simulink subsystem "Day3_Scenario_1"  (R2024a)
settings: Solver=VariableStepAuto  StartTime=0.0  StopTime=10.0  RelTol=1e-3
undefined symbols (not defined in the file): left_first_line_point_x, right_first_line_point_x
libraries: CarMaker4SL x6, slpidlib x1
settings Model: Creator=junhyung.cha  LastModifiedBy=User

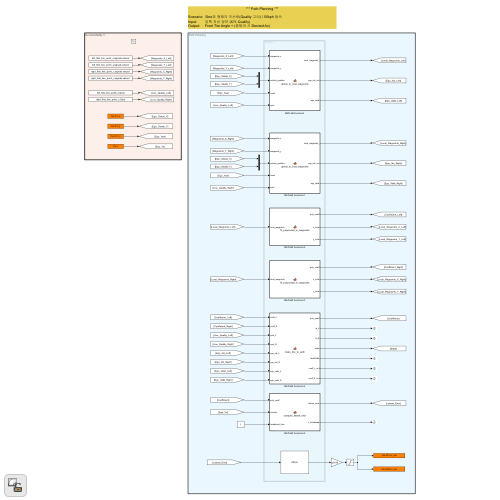
[thumbnail: Simulink's stored preview of the top-level diagram]
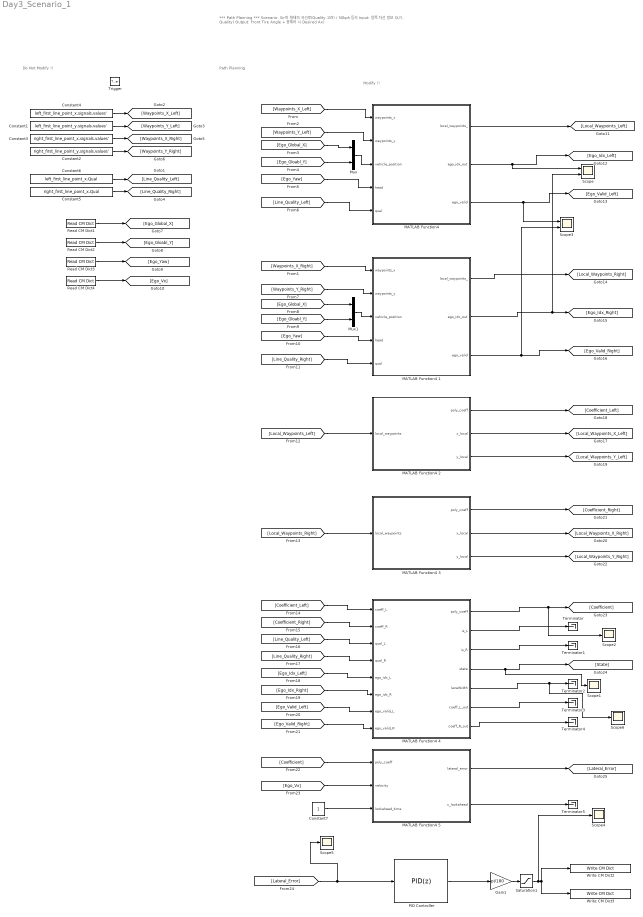
== system Day3_Scenario_1 ==
  note: Path Planning
  note: Do Not Modify !!
  note: Modify !!
  note: *** Path Planning ***
      |
      | Scenario: Sine파 형태의 곡선로(Quality 고려) / 50kph 등속
      | Input: 양쪽 차선 정보 (X/Y, Quality)
      | Output: Front Tire Angle + (종제어 시 Desired Ax)
  Trigger : TriggerPort  TriggerType=function-call  VariantControl=(inherit)
  Constant1 : Constant  Value=left_first_line_point_y.signals.values'
  Constant2 : Constant  Value=right_first_line_point_y.signals.values'
  Constant3 : Constant  Value=right_first_line_point_x.signals.values'
  Constant4 : Constant  Value=left_first_line_point_x.signals.values'
  Constant5 : Constant  Value=right_first_line_point_x.Qual
  Constant6 : Constant  Value=left_first_line_point_x.Qual
  Constant7 : Constant
  Gain1 : Gain  Gain=pi/180
  "MATLAB Function4 " : MATLAB Function  TreatAsAtomicUnit=on
  MATLAB Function4 1 : MATLAB Function  TreatAsAtomicUnit=on
  MATLAB Function4 2 : MATLAB Function  TreatAsAtomicUnit=on
  MATLAB Function4 3 : MATLAB Function  TreatAsAtomicUnit=on
  MATLAB Function4 4 : MATLAB Function  TreatAsAtomicUnit=on
  MATLAB Function4 5 : MATLAB Function  TreatAsAtomicUnit=on
  Mux : Mux  Inputs=2
  Mux1 : Mux  Inputs=2
  PID Controller : slpidlib/PID Controller  Controller=PID  Form=Parallel  TimeDomain=Discrete-time  UseExternalTs=off  SampleTime=-1  IntegratorMethod=Forward Euler  FilterMethod=Forward Euler  ControllerParametersSource=internal  P=0.2  I=0  UseKiTs=off  D=0.0001  UseExternalDerivativeSource=off  N=100  UseFilter=off  TunerSelectOption=Transfer Function Based (PID Tuner App)  InitialConditionSource=internal  InitialConditionForIntegrator=0  InitialConditionForFilter=0  DifferentiatorICPrevScaledInput=0  ExternalReset=none  TrackingMode=off  Kt=1  LimitOutput=off  SatLimitsSource=internal  UpperSaturationLimit=inf  LowerSaturationLimit=-inf  LinearizeAsGain=on  AntiWindupMode=none  Kb=1  LimitIntegrator=off  UpperIntegratorSaturationLimit=inf  LowerIntegratorSaturationLimit=-inf  POutMin=[]  POutMax=[]  IOutMin=[]  IOutMax=[]  DOutMin=[]  DOutMax=[]  NOutMin=[]  NOutMax=[]  SumOutMin=[]  SumOutMax=[]  SaturationOutMin=[]  SaturationOutMax=[]  PParamMin=[]  PParamMax=[]  IParamMin=[]  IParamMax=[]  DParamMin=[]  DParamMax=[]  NParamMin=[]  NParamMax=[]  KbParamMin=[]  KbParamMax=[]  KtParamMin=[]  KtParamMax=[]  KbOutMin=[]  KbOutMax=[]  KtOutMin=[]  KtOutMax=[]  IntegratorOutMin=[]  IntegratorOutMax=[]  FilterOutMin=[]  FilterOutMax=[]  SumI1OutMin=[]  SumI1OutMax=[]  SumI2OutMin=[]  SumI2OutMax=[]  SumI3OutMin=[]  SumI3OutMax=[]  SumI4OutMin=[]  SumI4OutMax=[]  SumDOutMin=[]  SumDOutMax=[]  DifferentiatorOutMin=[]  DifferentiatorOutMax=[]  FilterDiffOutCoefMin=[]  FilterDiffOutCoefMax=[]  ReciprocalOutMin=[]  ReciprocalOutMax=[]  SumDenOutMin=[]  SumDenOutMax=[]  SumNumOutMin=[]  SumNumOutMax=[]  DivideOutMin=[]  DivideOutMax=[]  UdiffTsProdOutMin=[]  UdiffTsProdOutMax=[]  NTsProdOutMin=[]  NTsProdOutMax=[]  UintegralTsProdOutMin=[]  UintegralTsProdOutMax=[]  UngainTsProdOutMin=[]  UngainTsProdOutMax=[]  ClampingZeroOutDataTypeStr=Inherit: Inherit via back propagation  ClampingZeroOutMin=[]  ClampingZeroOutMax=[]  FilterDenConstantOutDataTypeStr=Inherit: Inherit via back propagation  FilterDenConstantOutMin=[]  FilterDenConstantOutMax=[]  PCopyOutDataTypeStr=Inherit: Inherit via back propagation  PCopyOutMin=[]  PCopyOutMax=[]  NCopyOutDataTypeStr=Inherit: Inherit via back propagation  NCopyOutMin=[]  NCopyOutMax=[]  IntegratorContinuousStateAttributes=''  IntegratorStateMustResolveToSignalObject=off  IntegratorRTWStateStorageClass=Auto  FilterContinuousStateAttributes=''  FilterStateMustResolveToSignalObject=off  FilterRTWStateStorageClass=Auto  ParallelPVariant=InternalParameters  IdealPVariant=Disabled  IVariant=InternalParameters  DVariant=InternalParameters  IntegratorVariant=Discrete  SatVariant=Disabled  AWVariant=Passthrough  PCopyVariant=Disabled  TRVariant=Disabled  FdbkBlocksVariant=Forward  IdealPFdbkVariant=Disabled  SatFdbkVariant=Disabled  DerivativeFilterVariant=Differentiator  NVariant=Passthrough  NCopyVariant=Disabled_SignalSpec  FilterICVariant=InternalICsDifferentiator  IntegratorICVariant=InternalICs  ExternalResetVariant=Disabled  TRSumVariant=Passthrough  SumFdbkVariant=Disabled  SumVariant=Sum_PID  TsampFilterVariant=InternalTs  TsampNgainVariant=Passthrough  TsampIntegralVariant=Disabled_SignalSpec  ExternalSaturationOutDataTypeStr=Inherit: Same as second input  DerivativeSourceVariant=ErrorSignal
  Read CM Dict1 : CarMaker4SL/Read CM Dict  xname=Car.Fr1.tx  xsync=off  xstime=Inherited
  Read CM Dict2 : CarMaker4SL/Read CM Dict  xname=Car.Fr1.ty  xsync=off  xstime=Inherited
  Read CM Dict3 : CarMaker4SL/Read CM Dict  xname=Car.Fr1.rz  xsync=off  xstime=Inherited
  Read CM Dict4 : CarMaker4SL/Read CM Dict  xname=Car.v  xsync=off  xstime=Inherited
  Saturation1 : Saturate  UpperLimit=2  LowerLimit=-2
  Scope : Scope  NumInputPorts=2
  Scope{1..2,4..6} (5 alike) : Scope
  Scope3 : Scope  NumInputPorts=2
  Terminator{,1..5} (6 alike) : Terminator
  Write CM Dict2 : CarMaker4SL/Write CM Dict  xname=Car.CFL.rz_ext  xsync=off
  Write CM Dict3 : CarMaker4SL/Write CM Dict  xname=Car.CFR.rz_ext  xsync=off
  wires:
  Constant4/1 -> [Waypoints_X_Left]
  Constant1/1 -> [Waypoints_Y_Left]
  Constant2/1 -> [Waypoints_Y_Right]
  Constant3/1 -> [Waypoints_X_Right]
  [Waypoints_X_Left] -> "MATLAB Function4 "/1(waypoints_x)
  [Waypoints_Y_Left] -> "MATLAB Function4 "/2(waypoints_y)
  Mux/1 -> "MATLAB Function4 "/3(vehicle_position)
  [Ego_Global_X] -> Mux/1
  Read CM Dict2/1 -> [Ego_Gloabl_Y]
  Read CM Dict1/1 -> [Ego_Global_X]
  [Ego_Gloabl_Y] -> Mux/2
  Read CM Dict3/1 -> [Ego_Yaw]
  [Ego_Yaw] -> "MATLAB Function4 "/4(head)
  Constant5/1 -> [Line_Quality_Right]
  Constant6/1 -> [Line_Quality_Left]
  [Line_Quality_Right] -> MATLAB Function4 1/5(qual)
  [Ego_Yaw] -> MATLAB Function4 1/4(head)
  [Ego_Gloabl_Y] -> Mux1/2
  [Ego_Global_X] -> Mux1/1
  [Waypoints_Y_Right] -> MATLAB Function4 1/2(waypoints_y)
  [Waypoints_X_Right] -> MATLAB Function4 1/1(waypoints_x)
  Mux1/1 -> MATLAB Function4 1/3(vehicle_position)
  "MATLAB Function4 "/3(ego_valid) -> [Ego_Valid_Left], Scope3/1
  "MATLAB Function4 "/2(ego_idx_out) -> [Ego_Idx_Left], Scope/1
  "MATLAB Function4 "/1(local_waypoints_) -> [Local_Waypoints_Left]
  MATLAB Function4 1/1(local_waypoints_) -> [Local_Waypoints_Right]
  MATLAB Function4 1/2(ego_idx_out) -> [Ego_Idx_Right], Scope/2
  MATLAB Function4 1/3(ego_valid) -> [Ego_Valid_Right], Scope3/2
  [Local_Waypoints_Left] -> MATLAB Function4 2/1(local_waypoints)
  [Local_Waypoints_Right] -> MATLAB Function4 3/1(local_waypoints)
  MATLAB Function4 2/1(poly_coeff) -> [Coefficient_Left]
  MATLAB Function4 2/2(x_local) -> [Local_Waypoints_X_Left]
  MATLAB Function4 2/3(y_local) -> [Local_Waypoints_Y_Left]
  MATLAB Function4 3/3(y_local) -> [Local_Waypoints_Y_Right]
  MATLAB Function4 3/2(x_local) -> [Local_Waypoints_X_Right]
  MATLAB Function4 3/1(poly_coeff) -> [Coefficient_Right]
  [Coefficient_Left] -> MATLAB Function4 4/1(coeff_L)
  [Line_Quality_Left] -> MATLAB Function4 4/3(qual_L)
  [Ego_Idx_Left] -> MATLAB Function4 4/5(ego_idx_L)
  [Ego_Idx_Right] -> MATLAB Function4 4/6(ego_idx_R)
  [Ego_Valid_Left] -> MATLAB Function4 4/7(ego_valid_L)
  [Ego_Valid_Right] -> MATLAB Function4 4/8(ego_valid_R)
  MATLAB Function4 4/1(poly_coeff) -> [Coefficient], Scope2/1
  MATLAB Function4 4/4(state) -> [State], Scope1/1
  MATLAB Function4 4/2(is_L) -> Terminator/1
  MATLAB Function4 4/3(is_R) -> Terminator1/1
  MATLAB Function4 4/6(coeff_L_out) -> Terminator3/1
  MATLAB Function4 4/5(laneWidth) -> Terminator2/1, Scope6/1
  MATLAB Function4 4/7(coeff_R_out) -> Terminator4/1
  [Coefficient] -> MATLAB Function4 5/1(poly_coeff)
  Read CM Dict4/1 -> [Ego_Vx]
  [Ego_Vx] -> MATLAB Function4 5/2(velocity)
  Constant7/1 -> MATLAB Function4 5/3(lookahead_time)
  Saturation1/1 -> Write CM Dict3/1, Write CM Dict2/1, Scope4/1
  Gain1/1 -> Saturation1/1
  MATLAB Function4 5/1(lateral_error) -> [Lateral_Error]
  MATLAB Function4 5/2(x_lookahead) -> Terminator5/1
  [Lateral_Error] -> PID Controller/1, Scope5/1
  PID Controller/1 -> Gain1/1
  [Line_Quality_Left] -> "MATLAB Function4 "/5(qual)
  [Coefficient_Right] -> MATLAB Function4 4/2(coeff_R)
  [Line_Quality_Right] -> MATLAB Function4 4/4(qual_R)

== matlab function Day3_Scenario_1/MATLAB Function4 5 ==
  settings: sampleTime=0.1
  data: poly_coeff input; lateral_error output; x_lookahead output; velocity input; lookahead_time input
function [lateral_error, x_lookahead] = compute_lateral_error(poly_coeff, velocity, lookahead_time)
%#codegen
% compute_lateral_error - Look-ahead 지점에서의 lateral error 계산
%   poly_coeff     : 1x4 다항식 계수 [a3 a2 a1 a0]
%   velocity       : 차량 전진 속도 (m/s)
%   lookahead_time : look-ahead 시간 (s)
%
% 출력:
%   lateral_error  : lateral error + heading error 보정값
%   x_lookahead    : look-ahead 거리

    %% 1) lookahead 거리
    x_lookahead = velocity * lookahead_time;

    %% 2) 경로상의 y 위치
    y = polyval(poly_coeff, x_lookahead);

    %% 3) 경로 기울기 → 방향 각도
    dpoly = polyder(poly_coeff);
    dy_dx = polyval(dpoly, x_lookahead);
    path_theta = atan(dy_dx);

    %% 4) heading error (차량 방향 θ_vehicle = 0 가정)
    heading_error = path_theta;

    %% 5) lateral error 보정 (tunable gain)
    k_heading = 1.0;  
    lateral_error = y + k_heading * heading_error;
     %% 6) lateral error 클리핑 (안정성 확보)
    max_error = 10.0;  % 필요시 조절
    lateral_error = min(max(lateral_error, -max_error), max_error);
end

== matlab function Day3_Scenario_1/MATLAB Function4  ==
  settings: sampleTime=0.1
  data: waypoints_x input; waypoints_y input; local_waypoints_ output; vehicle_position input; head input; ego_idx_out output; ego_valid output; qual input
function [local_waypoints_, ego_idx_out, ego_valid] = global_to_local_waypoints_left(waypoints_x, waypoints_y, vehicle_position, head, qual)
    % 우측 차선 전역 → 로컬 좌표 변환 및 유효 인덱스 계산

    N = numel(waypoints_x);
    local_waypoints_ = zeros(N, 2);

    % 차량 yaw 방향의 회전 행렬 파라미터
    cos_h = cos(head);
    sin_h = sin(head);

    % 1) 전역 좌표 → 로컬 좌표
    for i = 1:N
        dx = waypoints_x(i) - vehicle_position(1);
        dy = waypoints_y(i) - vehicle_position(2);
        % (x', y') = R(-head) * [dx; dy]
        x_local =  dx * cos_h + dy * sin_h;
        y_local = -dx * sin_h + dy * cos_h;
        local_waypoints_(i, :) = [x_local, y_local];
    end

    % 2) qual == 1 (유효)인 인덱스들만 추출
    valid_indices = find(qual == 1);

    % 파라미터: 최대 인식 거리
    max_distance = 30; % meter

    % 3) 유효 지점 중 전방 x_local 거리 기준 최소값 선택 (30m 이내만)
    if ~isempty(valid_indices)
        x_vals = local_waypoints_(valid_indices, 1);
        d_vals = abs(x_vals);  % 전방 거리 기준
        d_vals(x_vals < 0 | d_vals > max_distance) = Inf;  % 후방 또는 너무 먼 점 제거

        [~, idx_min] = min(d_vals);
        if isinf(d_vals(idx_min))
            ego_idx_out = -1;
            ego_valid   = 0;
        else
            ego_idx_out = valid_indices(idx_min);
            ego_valid   = 1;
        end
    else
        ego_idx_out = -1;
        ego_valid   = 0;
    end
end

== matlab function Day3_Scenario_1/MATLAB Function4 1 ==
  settings: sampleTime=0.1
  data: waypoints_x input; waypoints_y input; local_waypoints_ output; vehicle_position input; head input; qual input; ego_idx_out output; ego_valid output
function [local_waypoints_, ego_idx_out, ego_valid] = global_to_local_waypoints_left(waypoints_x, waypoints_y, vehicle_position, head, qual)
    % 우측 차선 전역 → 로컬 좌표 변환 및 유효 인덱스 계산

    N = numel(waypoints_x);
    local_waypoints_ = zeros(N, 2);

    % 차량 yaw 방향의 회전 행렬 파라미터
    cos_h = cos(head);
    sin_h = sin(head);

    % 1) 전역 좌표 → 로컬 좌표
    for i = 1:N
        dx = waypoints_x(i) - vehicle_position(1);
        dy = waypoints_y(i) - vehicle_position(2);
        % (x', y') = R(-head) * [dx; dy]
        x_local =  dx * cos_h + dy * sin_h;
        y_local = -dx * sin_h + dy * cos_h;
        local_waypoints_(i, :) = [x_local, y_local];
    end

    % 2) qual == 1 (유효)인 인덱스들만 추출
    valid_indices = find(qual == 1);

    % 파라미터: 최대 인식 거리
    max_distance = 30; % meter

    % 3) 유효 지점 중 전방 x_local 거리 기준 최소값 선택 (30m 이내만)
    if ~isempty(valid_indices)
        x_vals = local_waypoints_(valid_indices, 1);
        d_vals = abs(x_vals);  % 전방 거리 기준
        d_vals(x_vals < 0 | d_vals > max_distance) = Inf;  % 후방 또는 너무 먼 점 제거

        [~, idx_min] = min(d_vals);
        if isinf(d_vals(idx_min))
            ego_idx_out = -1;
            ego_valid   = 0;
        else
            ego_idx_out = valid_indices(idx_min);
            ego_valid   = 1;
        end
    else
        ego_idx_out = -1;
        ego_valid   = 0;
    end
end

== matlab function Day3_Scenario_1/MATLAB Function4 2 ==
  settings: sampleTime=0.1
  data: local_waypoints input; poly_coeff output; x_local output; y_local output
function [poly_coeff, x_local, y_local] = fit_polynomial_to_waypoints(local_waypoints)
%#codegen
% Sliding-Window 기반 3차 다항식 피팅 (개선판)
%
% local_waypoints : Nx2 [x y] in vehicle-local frame
% poly_coeff      : 1x4 [a3 a2 a1 a0]
% x_local, y_local: MAX_POINTS×1 윈도우에 저장된 값 (나머지는 0)

    %% 파라미터
    MAX_DIST   = 15.0;    % 전방 최대 거리 [m]
    MAX_POINTS = 11;      % 최대 포인트 개수
    MAX_ORDER  = 3;       % 최대 다항식 차수

    %% 출력 초기화
    poly_coeff = zeros(1, MAX_ORDER+1);
    x_local    = zeros(MAX_POINTS,1);
    y_local    = zeros(MAX_POINTS,1);

    %% 1) 전방 필터링 + 윈도우 저장
    stored = 0;
    x_all = local_waypoints(:,1);
    y_all = local_waypoints(:,2);
    for i = 1:length(x_all)
        if x_all(i) > 0 && x_all(i) < MAX_DIST
            if stored < MAX_POINTS
                stored = stored + 1;
                x_local(stored) = x_all(i);
                y_local(stored) = y_all(i);
            end
        end
    end

    %% 2) 충분한 점 + 다양한 x 값 체크
    unique_x = numel(unique(x_local(1:stored)));
    if stored < 2 || unique_x < 2
        % 점이 너무 적거나 모두 같은 x → 피팅 불가
        return;
    end

    %% 3) 적정 차수 결정 (점 수에 따라 자동 축소)
    deg = min([MAX_ORDER, stored-1, unique_x-1]);

    %% 4) 정규화된 polyfit 호출
    %    mu = [mean(x), std(x)] 로 내부에서 정규화 처리
    [p, S, mu] = polyfit(x_local(1:stored), y_local(1:stored), deg);

    %% 5) 조건 수 확인 (optional)
    if isfield(S, 'R')
        condNum = cond(S.R);
        if condNum > 1e6
            % 너무 ill-conditioned → 낮은 차수 재시도
            deg = max(1, deg-1);
            [p, S, mu] = polyfit(x_local(1:stored), y_local(1:stored), deg);
        end
    end

    %% 6) 결과 확장 및 출력
    % p 는 [a_deg … a0] 길이 deg+1, 나머지 계수 0 패딩
    poly_coeff = zeros(1, MAX_ORDER+1);
    poly_coeff(end-deg:end) = p;

    % (추가) 만약 Eval 이 필요하면:
    % y_fit = polyval(p, x_query, S, mu);

end

== matlab function Day3_Scenario_1/MATLAB Function4 3 ==
  settings: sampleTime=0.1
  data: local_waypoints input; poly_coeff output; x_local output; y_local output
function [poly_coeff, x_local, y_local] = fit_polynomial_to_waypoints(local_waypoints)
%#codegen
% Sliding-Window 기반 3차 다항식 피팅 (개선판)
%
% local_waypoints : Nx2 [x y] in vehicle-local frame
% poly_coeff      : 1x4 [a3 a2 a1 a0]
% x_local, y_local: MAX_POINTS×1 윈도우에 저장된 값 (나머지는 0)

    %% 파라미터
    MAX_DIST   = 15.0;    % 전방 최대 거리 [m]
    MAX_POINTS = 11;      % 최대 포인트 개수
    MAX_ORDER  = 3;       % 최대 다항식 차수

    %% 출력 초기화
    poly_coeff = zeros(1, MAX_ORDER+1);
    x_local    = zeros(MAX_POINTS,1);
    y_local    = zeros(MAX_POINTS,1);

    %% 1) 전방 필터링 + 윈도우 저장
    stored = 0;
    x_all = local_waypoints(:,1);
    y_all = local_waypoints(:,2);
    for i = 1:length(x_all)
        if x_all(i) > 0 && x_all(i) < MAX_DIST
            if stored < MAX_POINTS
                stored = stored + 1;
                x_local(stored) = x_all(i);
                y_local(stored) = y_all(i);
            end
        end
    end

    %% 2) 충분한 점 + 다양한 x 값 체크
    unique_x = numel(unique(x_local(1:stored)));
    if stored < 2 || unique_x < 2
        % 점이 너무 적거나 모두 같은 x → 피팅 불가
        return;
    end

    %% 3) 적정 차수 결정 (점 수에 따라 자동 축소)
    deg = min([MAX_ORDER, stored-1, unique_x-1]);

    %% 4) 정규화된 polyfit 호출
    %    mu = [mean(x), std(x)] 로 내부에서 정규화 처리
    [p, S, mu] = polyfit(x_local(1:stored), y_local(1:stored), deg);

    %% 5) 조건 수 확인 (optional)
    if isfield(S, 'R')
        condNum = cond(S.R);
        if condNum > 1e6
            % 너무 ill-conditioned → 낮은 차수 재시도
            deg = max(1, deg-1);
            [p, S, mu] = polyfit(x_local(1:stored), y_local(1:stored), deg);
        end
    end

    %% 6) 결과 확장 및 출력
    % p 는 [a_deg … a0] 길이 deg+1, 나머지 계수 0 패딩
    poly_coeff = zeros(1, MAX_ORDER+1);
    poly_coeff(end-deg:end) = p;

    % (추가) 만약 Eval 이 필요하면:
    % y_fit = polyval(p, x_query, S, mu);

end

== matlab function Day3_Scenario_1/MATLAB Function4 4 ==
  settings: sampleTime=0.1
  data: coeff_L input; coeff_R input; poly_coeff output; is_L output; is_R output; qual_L input; qual_R input; ego_idx_L input; ego_idx_R input; ego_valid_L input; state output; laneWidth output; coeff_L_out output; ego_valid_R input; coeff_R_out output
function [poly_coeff, is_L, is_R, state, laneWidth, coeff_L_out, coeff_R_out] = ...
         make_line_to_path(coeff_L, coeff_R, qual_L, qual_R, ...
                           ego_idx_L, ego_idx_R, ego_valid_L, ego_valid_R)
%#codegen
% 양쪽/한쪽 차선에 따라 center path를 만드는 함수
% 
% 입력:
%  coeff_L/R    : 1x4 [a3 a2 a1 a0]
%  ego_valid_L/R: 좌/우 유효 플래그 (0/1)
%
% 출력:
%  poly_coeff   : 1x4 center path coeff
%  is_L, is_R   : 입력 플래그 그대로
%  state        : 1=both,2=left only,3=right only,4=width invalid,0=none
%  laneWidth    : 최종 차폭 (m)
%  coeff_L_out  : 실제 사용된 left coeff (원본 or synthetic)
%  coeff_R_out  : 실제 사용된 right coeff

  persistent prev_laneWidth prev_coeff_L prev_coeff_R prev_state
  if isempty(prev_laneWidth)
    prev_laneWidth = 3.5;             % 초기 추정 차폭 (m)
    prev_coeff_L   = zeros(1,4);
    prev_coeff_R   = zeros(1,4);
    prev_state     = 0;
  end

  %--- 파라미터 ---%
  alpha       = 0.3;    % 차폭 EMA 계수
  minWidth    = 2.0;    % 최소 허용 차폭 (m)
  maxWidth    = 5.0;    % 최대 허용 차폭 (m)

  %--- 플래그 복사 ---%
  is_L = ego_valid_L;
  is_R = ego_valid_R;

  %--- 케이스 분기 ---%
  if is_L && is_R
    % 1) 양쪽 다 보일 때 → 차폭 계산 & EMA
    rawWidth = abs(coeff_L(4) - coeff_R(4));
    if rawWidth >= minWidth && rawWidth <= maxWidth
      laneWidth = alpha*rawWidth + (1-alpha)*prev_laneWidth;
      state     = 1;
    else
      % 폭이 터무니없으면 이전 값 유지
      laneWidth = prev_laneWidth;
      state     = 4;
    end
    coeff_L_out = coeff_L;
    coeff_R_out = coeff_R;

  elseif is_L
    % 2) 왼쪽만 보일 때 → synthetic right
    laneWidth   = prev_laneWidth;
    coeff_L_out = coeff_L;
    coeff_R_out = coeff_L;                % 곡률 그대로 복사
    coeff_R_out(4) = coeff_R_out(4) - laneWidth;
    state       = 2;

  elseif is_R
    % 3) 오른쪽만 보일 때 → synthetic left
    laneWidth   = prev_laneWidth;
    coeff_R_out = coeff_R;
    coeff_L_out = coeff_R;
    coeff_L_out(4) = coeff_L_out(4) + laneWidth;
    state       = 3;

  else
    % 4) 둘 다 없을 때 → 이전 값 유지
    laneWidth   = prev_laneWidth;
    coeff_L_out = prev_coeff_L;
    coeff_R_out = prev_coeff_R;
    state       = prev_state;
  end

  %--- center path 다항식 (항상 두 계수의 평균) ---%
  poly_coeff = (coeff_L_out + coeff_R_out) * 0.5;

  %--- persistent 업데이트 ---%
  prev_laneWidth = laneWidth;
  % prev_coeff_L   = coeff_L_out;
  % prev_coeff_R   = coeff_R_out;
  prev_state     = state;
end
